simulink model "TST_MeUn_Rot"  (R2016b)
settings: Solver=FixedStepDiscrete  StartTime=0.0  StopTime=simTime  FixedStep=sampleTime  RelTol=1e-3
values from neighbouring files (symbols this model uses):
  testCase = 1    [initTST_MeUn_Rot_001.m]
libraries: simulink x4, UnitTest_Lib x2
settings Model: Creator=zhengjinyan  LastModifiedBy=zhengjinyan
settings DebuggingCC: SignalRangeChecking=error

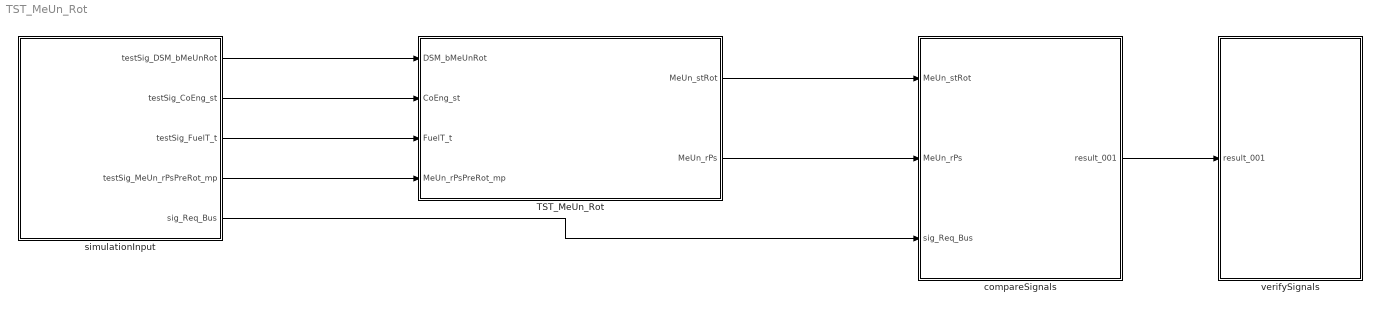
== system TST_MeUn_Rot ==
  TST_MeUn_Rot : Subsystem
  compareSignals : Subsystem
  simulationInput : Subsystem
  verifySignals : Subsystem
  wires:
  simulationInput/1(testSig_DSM_bMeUnRot) -> TST_MeUn_Rot/1(DSM_bMeUnRot)
  simulationInput/2(testSig_CoEng_st) -> TST_MeUn_Rot/2(CoEng_st)
  simulationInput/3(testSig_FuelT_t) -> TST_MeUn_Rot/3(FuelT_t)
  simulationInput/4(testSig_MeUn_rPsPreRot_mp) -> TST_MeUn_Rot/4(MeUn_rPsPreRot_mp)
  TST_MeUn_Rot/1(MeUn_stRot) -> compareSignals/1(MeUn_stRot)
  TST_MeUn_Rot/2(MeUn_rPs) -> compareSignals/2(MeUn_rPs)
  simulationInput/5(sig_Req_Bus) -> compareSignals/3(sig_Req_Bus)
  compareSignals/1(result_001) -> verifySignals/1(result_001)

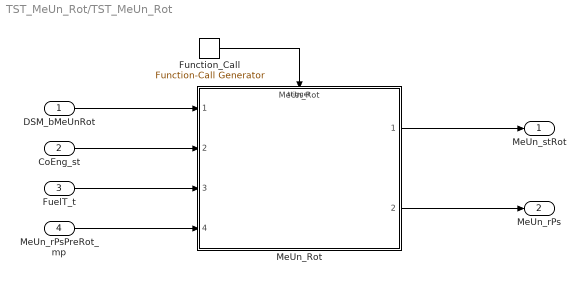
== system TST_MeUn_Rot/TST_MeUn_Rot ==
  DSM_bMeUnRot : Inport
  CoEng_st : Inport  Port=2
  FuelT_t : Inport  Port=3
  MeUn_rPsPreRot_mp : Inport  Port=4
  Function_Call : simulink/Ports & Subsystems/Function-Call Generator  sample_time=sampleTime  numberOfIterations=1
  MeUn_Rot : ModelReference  ModelNameDialog=MeUn_Rot  SimulationMode=Normal  ModelReferenceVersion=1.6  TriggerPortName=function  TriggerPortTriggerType=function-call  TriggerPortStatesWhenEnabling=held
  MeUn_stRot : Outport
  MeUn_rPs : Outport  Port=2
  wires:
  Function_Call/1 -> MeUn_Rot/Trigger
  DSM_bMeUnRot/1 -> MeUn_Rot/1
  CoEng_st/1 -> MeUn_Rot/2
  FuelT_t/1 -> MeUn_Rot/3
  MeUn_rPsPreRot_mp/1 -> MeUn_Rot/4
  MeUn_Rot/1 -> MeUn_stRot/1
  MeUn_Rot/2 -> MeUn_rPs/1

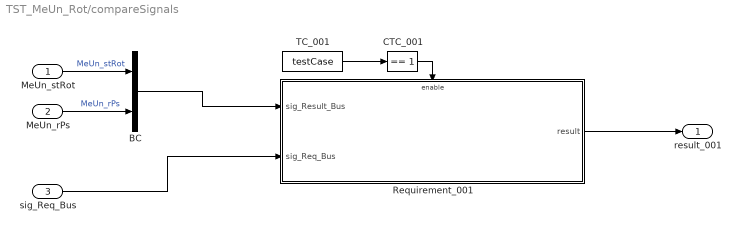
== system TST_MeUn_Rot/compareSignals ==
  MeUn_stRot : Inport
  MeUn_rPs : Inport  Port=2
  sig_Req_Bus : Inport  Port=3
  BC : BusCreator  Inputs=2
  CTC_001 : simulink/Logic and Bit Operations/Compare To Constant  relop===  const=1  OutDataTypeStr=boolean
  Requirement_001 : Subsystem
  TC_001 : Constant  Value=testCase
  result_001 : Outport
  wires:
  MeUn_stRot/1 -> BC/1  "MeUn_stRot"
  MeUn_rPs/1 -> BC/2  "MeUn_rPs"
  TC_001/1 -> CTC_001/1
  CTC_001/1 -> Requirement_001/Enable
  sig_Req_Bus/1 -> Requirement_001/2(sig_Req_Bus)
  BC/1 -> Requirement_001/1(sig_Result_Bus)
  Requirement_001/1(result) -> result_001/1

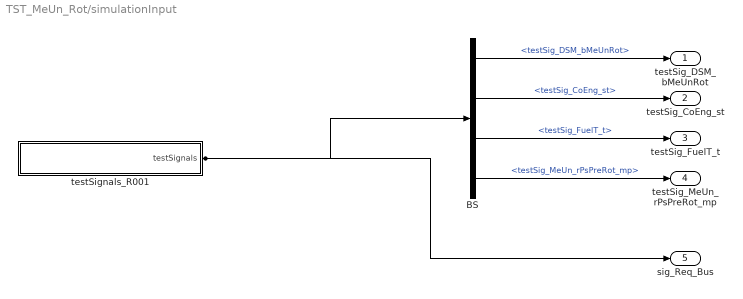
== system TST_MeUn_Rot/simulationInput ==
  BS : BusSelector  OutputSignals=testSig_DSM_bMeUnRot,testSig_CoEng_st,testSig_FuelT_t,testSig_MeUn_rPsPreRot_mp
  testSignals_R001 : Subsystem
  testSig_DSM_bMeUnRot : Outport
  testSig_CoEng_st : Outport  Port=2
  testSig_FuelT_t : Outport  Port=3
  testSig_MeUn_rPsPreRot_mp : Outport  Port=4
  sig_Req_Bus : Outport  Port=5
  wires:
  BS/1 -> testSig_DSM_bMeUnRot/1  "<testSig_DSM_bMeUnRot>"
  BS/2 -> testSig_CoEng_st/1  "<testSig_CoEng_st>"
  BS/3 -> testSig_FuelT_t/1  "<testSig_FuelT_t>"
  BS/4 -> testSig_MeUn_rPsPreRot_mp/1  "<testSig_MeUn_rPsPreRot_mp>"
  testSignals_R001/1(testSignals) -> BS/1, sig_Req_Bus/1

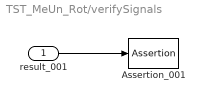
== system TST_MeUn_Rot/verifySignals ==
  result_001 : Inport
  Assertion_001 : Assertion  Enabled=off
  wires:
  result_001/1 -> Assertion_001/1

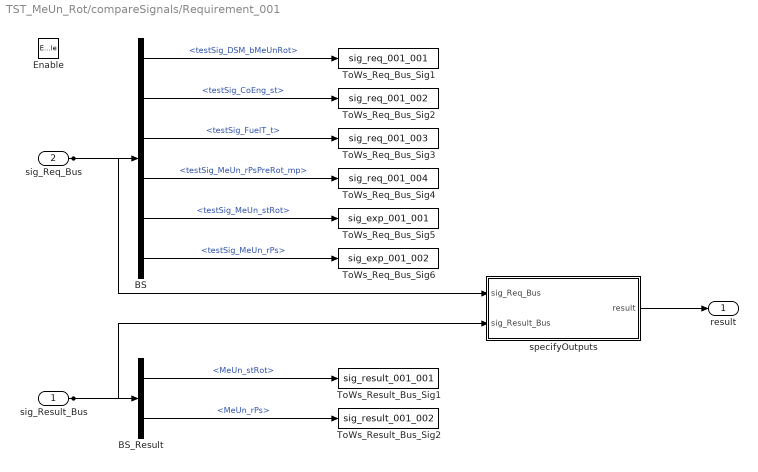
== system TST_MeUn_Rot/compareSignals/Requirement_001 ==
  sig_Result_Bus : Inport
  sig_Req_Bus : Inport  Port=2
  Enable : EnablePort
  BS : BusSelector  OutputSignals=testSig_DSM_bMeUnRot,testSig_CoEng_st,testSig_FuelT_t,testSig_MeUn_rPsPreRot_mp,testSig_MeUn_stRot,testSig_MeUn_rPs
  BS_Result : BusSelector  OutputSignals=MeUn_stRot,MeUn_rPs
  ToWs_Req_Bus_Sig1 : ToWorkspace  VariableName=sig_req_001_001  SaveFormat=Structure With Time
  ToWs_Req_Bus_Sig2 : ToWorkspace  VariableName=sig_req_001_002  SaveFormat=Structure With Time
  ToWs_Req_Bus_Sig3 : ToWorkspace  VariableName=sig_req_001_003  SaveFormat=Structure With Time
  ToWs_Req_Bus_Sig4 : ToWorkspace  VariableName=sig_req_001_004  SaveFormat=Structure With Time
  ToWs_Req_Bus_Sig5 : ToWorkspace  VariableName=sig_exp_001_001  SaveFormat=Structure With Time
  ToWs_Req_Bus_Sig6 : ToWorkspace  VariableName=sig_exp_001_002  SaveFormat=Structure With Time
  ToWs_Result_Bus_Sig1 : ToWorkspace  VariableName=sig_result_001_001  SaveFormat=Structure With Time
  ToWs_Result_Bus_Sig2 : ToWorkspace  VariableName=sig_result_001_002  SaveFormat=Structure With Time
  specifyOutputs : Subsystem
  result : Outport
  wires:
  sig_Req_Bus/1 -> BS/1, specifyOutputs/1(sig_Req_Bus)
  BS/1 -> ToWs_Req_Bus_Sig1/1  "<testSig_DSM_bMeUnRot>"
  BS/2 -> ToWs_Req_Bus_Sig2/1  "<testSig_CoEng_st>"
  BS/3 -> ToWs_Req_Bus_Sig3/1  "<testSig_FuelT_t>"
  BS/4 -> ToWs_Req_Bus_Sig4/1  "<testSig_MeUn_rPsPreRot_mp>"
  BS/5 -> ToWs_Req_Bus_Sig5/1  "<testSig_MeUn_stRot>"
  BS/6 -> ToWs_Req_Bus_Sig6/1  "<testSig_MeUn_rPs>"
  sig_Result_Bus/1 -> BS_Result/1, specifyOutputs/2(sig_Result_Bus)
  BS_Result/1 -> ToWs_Result_Bus_Sig1/1  "<MeUn_stRot>"
  BS_Result/2 -> ToWs_Result_Bus_Sig2/1  "<MeUn_rPs>"
  specifyOutputs/1(result) -> result/1

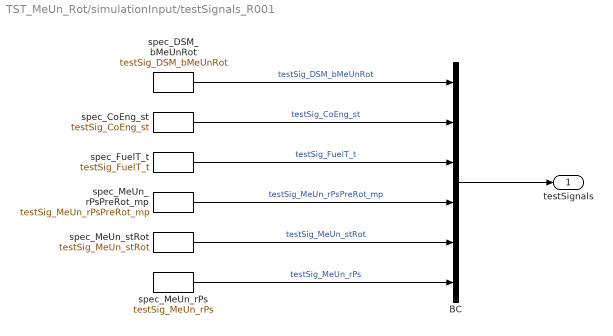
== system TST_MeUn_Rot/simulationInput/testSignals_R001 ==
  BC : BusCreator  Inputs=6
  spec_CoEng_st : FromWorkspace  VariableName=testSig_CoEng_st  Interpolate=off  OutputAfterFinalValue=Holding final value
  spec_DSM_bMeUnRot : FromWorkspace  VariableName=testSig_DSM_bMeUnRot  Interpolate=off  OutputAfterFinalValue=Holding final value
  spec_FuelT_t : FromWorkspace  VariableName=testSig_FuelT_t  Interpolate=off  OutputAfterFinalValue=Holding final value
  spec_MeUn_rPs : FromWorkspace  VariableName=testSig_MeUn_rPs  Interpolate=off  OutputAfterFinalValue=Holding final value
  spec_MeUn_rPsPreRot_mp : FromWorkspace  VariableName=testSig_MeUn_rPsPreRot_mp  Interpolate=off  OutputAfterFinalValue=Holding final value
  spec_MeUn_stRot : FromWorkspace  VariableName=testSig_MeUn_stRot  Interpolate=off  OutputAfterFinalValue=Holding final value
  testSignals : Outport
  wires:
  BC/1 -> testSignals/1
  spec_DSM_bMeUnRot/1 -> BC/1  "testSig_DSM_bMeUnRot"
  spec_CoEng_st/1 -> BC/2  "testSig_CoEng_st"
  spec_FuelT_t/1 -> BC/3  "testSig_FuelT_t"
  spec_MeUn_rPsPreRot_mp/1 -> BC/4  "testSig_MeUn_rPsPreRot_mp"
  spec_MeUn_stRot/1 -> BC/5  "testSig_MeUn_stRot"
  spec_MeUn_rPs/1 -> BC/6  "testSig_MeUn_rPs"

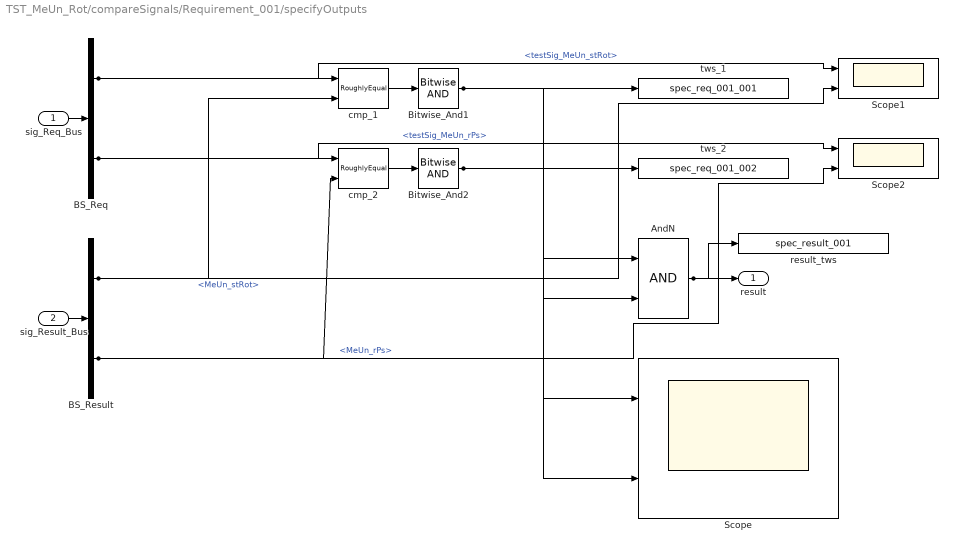
== system TST_MeUn_Rot/compareSignals/Requirement_001/specifyOutputs ==
  sig_Req_Bus : Inport
  sig_Result_Bus : Inport  Port=2
  AndN : Logic
  BS_Req : BusSelector  OutputSignals=testSig_MeUn_stRot,testSig_MeUn_rPs
  BS_Result : BusSelector  OutputSignals=MeUn_stRot,MeUn_rPs
  Bitwise_And1 : simulink/Logic and Bit Operations/Bitwise Operator  logicop=AND  UseBitMask=off  BitMask=bin2dec('11011001')  BitMaskRealWorld=Stored Integer
  Bitwise_And2 : simulink/Logic and Bit Operations/Bitwise Operator  logicop=AND  UseBitMask=off  BitMask=bin2dec('11011001')  BitMaskRealWorld=Stored Integer
  Scope : Scope  NumInputPorts=2
  Scope1 : Scope  NumInputPorts=2
  Scope2 : Scope  NumInputPorts=2
  cmp_1 : UnitTest_Lib/RoughlyEqual  slope=0.1
  cmp_2 : UnitTest_Lib/RoughlyEqual  slope=0.1
  result_tws : ToWorkspace  VariableName=spec_result_001
  tws_1 : ToWorkspace  VariableName=spec_req_001_001
  tws_2 : ToWorkspace  VariableName=spec_req_001_002
  result : Outport
  wires:
  sig_Req_Bus/1 -> BS_Req/1
  sig_Result_Bus/1 -> BS_Result/1
  AndN/1 -> result/1, result_tws/1
  BS_Req/1 -> cmp_1/1, Scope1/1  "<testSig_MeUn_stRot>"
  BS_Result/1 -> cmp_1/2, Scope1/2  "<MeUn_stRot>"
  cmp_1/1 -> Bitwise_And1/1
  Bitwise_And1/1 -> tws_1/1, AndN/1, Scope/1
  BS_Req/2 -> cmp_2/1, Scope2/1  "<testSig_MeUn_rPs>"
  BS_Result/2 -> cmp_2/2, Scope2/2  "<MeUn_rPs>"
  cmp_2/1 -> Bitwise_And2/1
  Bitwise_And2/1 -> tws_2/1, AndN/2, Scope/2
